simulink model "moment_udarowy"  (R2021b)
settings: Solver=ode45  StartTime=0.0  StopTime=15  MaxStep=0.001  MinStep=0.0001  RelTol=1e-3
values from neighbouring files (symbols this model uses):
  In = 88    [P.m]    (also in PI.m; faza.m)
  J = 22*Js    (= 6.05)    [P.m]    (also in PI.m; faza.m)
  Kp = 1.5*Un/10    (= 33)    [P.m]    (also in PI.m; faza.m)
  Kt = 10/(1.2*wn)    (= 0.0530516476973)    [P.m]    (also in PI.m; faza.m)
  Kw = Mm/(psi_e*kz*Kt*dw*wn)    [P.m]    (also in PI.m = J/(2*Kt*kz*Beta*psi_e); faza.m = J/(2*Kt*kz*Beta*psi_e))
  lambda_n = 5    [P.m]    (also in PI.m = 2; faza.m = 2)
  m = T1    [P.m]    (also in PI.m; faza.m)
  Mn = psi_e*In    (= 115.854612655)    [P.m]    (also in PI.m; faza.m)
  psi_e = (Un-In*R)/wn    (= 1.31652968926)    [P.m]    (also in PI.m; faza.m)
  R = Rt    (= 0.15)    [P.m]    (also in PI.m; faza.m)
  T = L/R    (= 0.125)    [P.m]    (also in PI.m; faza.m)
  TR = 4*Beta    (= 0.16)    [PI.m]    (also in faza.m)
  Uz0 = 0.937*lambda_n*In*Y*B1/(B1-Beta)    [P.m]    (also in PI.m; faza.m)
  V = Beta*Y*Kp*B/((B1-Beta)*Rt)    [P.m]    (also in PI.m; faza.m)
  wz = wn*Kt    (= 8.33333333333)    [P.m]    (also in PI.m; faza.m)
  Y = 10/(2.5*In)    (= 0.0454545454545)    [P.m]    (also in PI.m; faza.m)
libraries: spspowerguiLib x1
settings Model: Creator=Admin  LastModifiedBy=gabrys
settings SolverCC: AlgebraicLoopSolver=TrustRegion
settings DataIOCC: LimitDataPoints=on  SaveFormat=Array  SignalLoggingSaveFormat=ModelDataLogs  ReturnWorkspaceOutputs=off
settings OptimizationCC: BlockReduction=off  BooleanDataType=off  LifeSpan=inf
settings DebuggingCC: SaveWithParameterizedLinksMsg=none  UnderspecifiedInitializationDetection=Classic  MergeDetectMultiDrivingBlocksExec=none  SignalResolutionControl=TryResolveAllWithWarning  MultiTaskDSMMsg=warning  MultiTaskCondExecSysMsg=none  StateNameClashWarn=warning  SFUnexpectedBacktrackingDiag=warning  SFNoUnconditionalDefaultTransitionDiag=warning  SFExecutionAtInitializationDiag=none  SFMachineParentedDataDiag=warning  ArithmeticOperatorsInVariantConditions=warning
settings HardwareCC: ProdBitPerPointer=32  ProdBitPerSizeT=32  ProdBitPerPtrDiffT=32  ProdLargestAtomicFloat=None  ProdIntDivRoundTo=Undefined  ProdEndianess=Unspecified  ProdWordSize=32  ProdHWDeviceType=32-bit Generic  TargetUnknown=on
settings ModelReferenceCC: PropagateSignalLabelsOutOfModel=off
settings SFSimCC: SimUseLocalCustomCode=off  CustomCodeUndefinedFunction=UseInterfaceOnly
settings RTWCC: RTWUseLocalCustomCode=off  DLArmComputeVersion=20.02.1
settings CodeAppCC: StateflowObjectComments=on
settings GRTTargetCC: TargetLangStandard=C89/C90 (ANSI)
settings ConfigComp: CovMetricSettings=dw  CovSaveCumulativeToWorkspaceVar=on  CovSaveSingleToWorkspaceVar=on  CovExternalEMLEnable=off

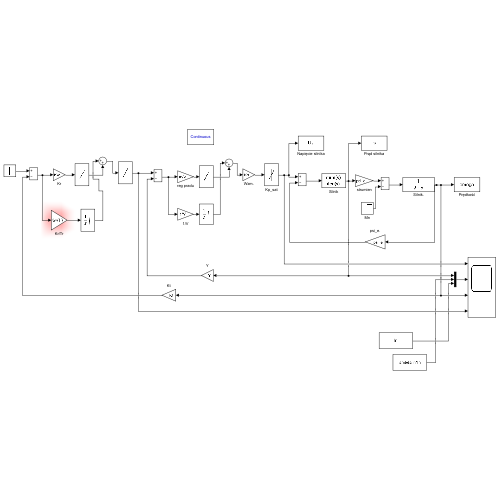
[thumbnail: Simulink's stored preview of the top-level diagram]
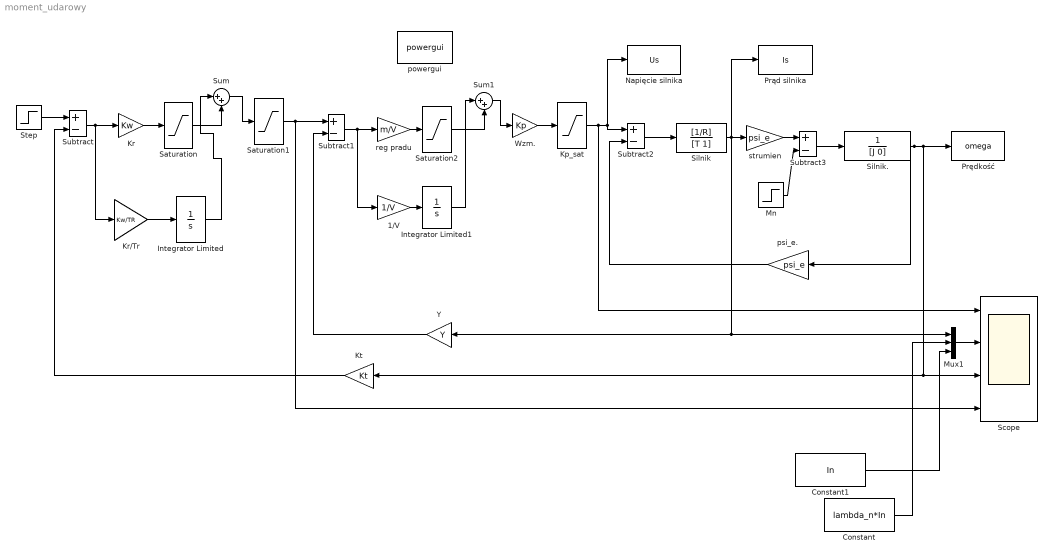
== system moment_udarowy ==
  1/V : Gain  Gain=1/V
  Constant : Constant  Value=lambda_n*In
  Constant1 : Constant  Value=In
  Integrator Limited : Integrator  LimitOutput=on  UpperSaturationLimit=10  LowerSaturationLimit=-10
  Integrator Limited1 : Integrator  LimitOutput=on  UpperSaturationLimit=10  LowerSaturationLimit=-10
  Kp_sat : Saturate  UpperLimit=500  LowerLimit=-500
  Kr : Gain  Gain=Kw
  Kr/Tr : Gain  Gain=Kw/TR
  Kt : Gain  Gain=Kt
  Mn : Step  Time=9  After=Mn  SampleTime=0
  Mux1 : Mux  Inputs=3
  Napięcie silnika : ToWorkspace  VariableName=Us  SaveFormat=Structure With Time  SampleTime=-1
  Prąd silnika : ToWorkspace  VariableName=Is  SaveFormat=Structure With Time  SampleTime=-1
  Prędkość : ToWorkspace  VariableName=omega  SaveFormat=Structure With Time  SampleTime=-1
  Saturation : Saturate  UpperLimit=10  LowerLimit=-10
  Saturation1 : Saturate  UpperLimit=Uz0  LowerLimit=-Uz0
  Saturation2 : Saturate  UpperLimit=10  LowerLimit=-10
  Scope : Scope  NumInputPorts=4
  Silnik : TransferFcn  Numerator=[1/R]  Denominator=[T 1]
  Silnik. : TransferFcn  Denominator=[J 0]
  Step : Step  Time=0  After=wz  SampleTime=0
  Subtract{,1..3} (4 alike) : Sum  Inputs=+-
  Sum : Sum  Inputs=|++
  Sum1 : Sum  Inputs=|++
  Wzm. : Gain  Gain=Kp
  Y : Gain  Gain=Y
  powergui : spspowerguiLib/powergui  Priority=1  SimulationMode=Continuous  SampleTime=50e-6  frequency=60  Iterations=50  frequencyindice=60  Pbase=100e6  ErrMax=1e-4  UnitsV=kV  UnitsW=MW  buscounter=0  FunctionMessages=off  echomessages=off  EnableUseOfTLC=off  CurrentSourceSwitches=on  DisableSnubberDevices=off  DisableRonSwitches=off  DisableVfSwitches=off  DisplayEquations=off  AutomaticDiscreteSolvers=off  SolverType=Tustin  Interpol=off  ExternalGateDelay=off  methode=off  Ts=0  x0status=blocks  SPID=off  SwTol=0  HookPort=off  NonlinearTolerance=1e-4  nMaxIteration=100  ContinueOnMaxIteration=off  RestoreLinks=warning  ResistiveCurrentMeasurement=off  Frange=[0:2:500]  Ylog=off  Xlog=on  ShowGrid=off  save=off  variable=ZData  structure=0  ZoomFFT=off  StartTime=0.0  cycles=1  DisplayStyle=1  fundamental=60  FreqAxis=off  MaxFrequency=1000  frequencyindicesteady=1  RmsSteady=1  display=off
  psi_e. : Gain  Gain=psi_e
  reg pradu : Gain  Gain=m/V
  strumien : Gain  Gain=psi_e
  wires:
  Step/1 -> Subtract/1
  Kr/1 -> Saturation/1
  Subtract/1 -> Kr/Tr/1, Kr/1
  Kr/Tr/1 -> Integrator Limited/1
  Saturation1/1 -> Scope/4, Subtract1/1
  Subtract1/1 -> 1/V/1, reg pradu/1
  reg pradu/1 -> Saturation2/1
  1/V/1 -> Integrator Limited1/1
  Sum1/1 -> Wzm./1
  Wzm./1 -> Kp_sat/1
  Kp_sat/1 -> Scope/1, Subtract2/1, Napięcie silnika/1
  Subtract2/1 -> Silnik/1
  Silnik/1 -> strumien/1, Prąd silnika/1, Mux1/1, Y/1
  strumien/1 -> Subtract3/1
  Subtract3/1 -> Silnik./1
  Mn/1 -> Subtract3/2
  psi_e./1 -> Subtract2/2
  Y/1 -> Subtract1/2
  Kt/1 -> Subtract/2
  Silnik./1 -> psi_e./1, Kt/1, Scope/3, Prędkość/1
  Constant/1 -> Mux1/2
  Saturation/1 -> Sum/2
  Integrator Limited/1 -> Sum/1
  Sum/1 -> Saturation1/1
  Integrator Limited1/1 -> Sum1/1
  Saturation2/1 -> Sum1/2
  Mux1/1 -> Scope/2
  Constant1/1 -> Mux1/3
